simulink model "filters"  (R2025b)
settings: Solver=FixedStepDiscrete  StartTime=0.0  StopTime=inf  RelTol=1e-3
undefined symbols (not defined in the file or in its folder): Gain_rt
settings Model: Creator=linogarciamorales  LastModifiedBy=linogarciamorales
settings OptimizationCC: EnhancedBackFolding=on  PassReuseOutputArgsAs=Individual arguments  ZeroExternalMemoryAtStartup=off  ZeroInternalMemoryAtStartup=off  OptimizeBlockOrder=speed  DifferentSizesBufferReuse=on  OptimizationCustomize=off  EfficientTunableParamExpr=on
settings DebuggingCC: ParameterTunabilityLossMsg=error
settings HardwareCC: ProdBitPerPointer=32.0  ProdBitPerSizeT=32.0  ProdBitPerPtrDiffT=32.0  ProdLargestAtomicFloat=None  ProdIntDivRoundTo=Undefined  ProdEndianess=Unspecified  ProdWordSize=32.0  ProdHWDeviceType=Generic->32-bit Embedded Processor
settings SFSimCC: MATLABDynamicMemAlloc=off
settings RTWCC: SystemTargetFile=ert.tlc  GenCodeOnly=on  TemplateMakefile=ert_default_tmf  Description=Embedded Coder
settings CodeAppCC: ForceParamTrailComments=on  IgnoreCustomStorageClasses=off  OperatorAnnotations=on  SimulinkDataObjDesc=on  SFDataObjDesc=on  InsertBlockDesc=on
settings ERTTargetCC: InlinedParameterPlacement=Hierarchical  ERTCustomFileTemplate=example_file_process.tlc  TargetLangStandard=C99 (ISO)  SupportNonInlinedSFcns=on

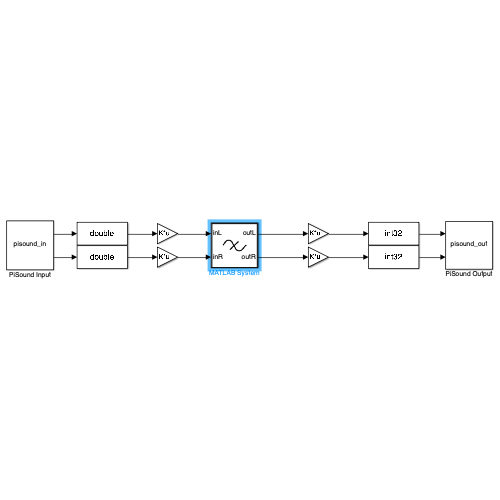
[thumbnail: Simulink's stored preview of the top-level diagram]
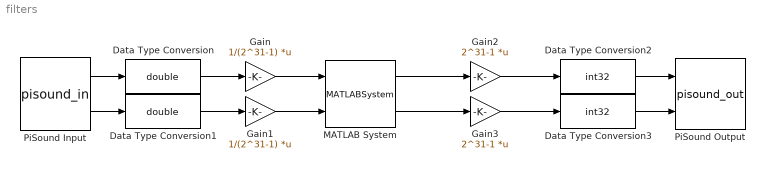
== system filters ==
  Data Type Conversion : DataTypeConversion  OutDataTypeStr=double  SaturateOnIntegerOverflow=off  RndMeth=Floor
  Data Type Conversion1 : DataTypeConversion  OutDataTypeStr=double  SaturateOnIntegerOverflow=off  RndMeth=Floor
  Data Type Conversion2 : DataTypeConversion  OutDataTypeStr=int32  SaturateOnIntegerOverflow=off  RndMeth=Floor
  Data Type Conversion3 : DataTypeConversion  OutDataTypeStr=int32  SaturateOnIntegerOverflow=off  RndMeth=Floor
  Gain : Gain  Gain=1/(2^31-1)  Multiplication=Matrix(K*u)
  Gain1 : Gain  Gain=1/(2^31-1)  Multiplication=Matrix(K*u)
  Gain2 : Gain  Gain=2^31-1  Multiplication=Matrix(K*u)
  Gain3 : Gain  Gain=2^31-1  Multiplication=Matrix(K*u)
  MATLAB System : MATLABSystem  InitFcn=|  System=filters_sys  N=128  Fs=48000  FilterType=FilterType_rt  Freq=Freq_rt  Q=Q_rt  Gain=Gain_rt  SimulateUsing=Code generation
      | Type_rt = uint8(1);   % 1..7
      | Freq_rt = 1000;       % Hz
      | Q_rt    = 0.707;
      | Gain_rt = 0;          % dB
      mask Type: filters_sys
  PiSound Input : S-Function  FunctionName=pisound_in  Parameters=48000, 128, 0  SFunctionDeploymentMode=off  EnableBusSupport=off
  PiSound Output : S-Function  FunctionName=pisound_out  Parameters=48000, 128, 0  SFunctionDeploymentMode=off  EnableBusSupport=off
  wires:
  PiSound Input/1 -> Data Type Conversion/1
  PiSound Input/2 -> Data Type Conversion1/1
  Data Type Conversion/1 -> Gain/1
  Data Type Conversion1/1 -> Gain1/1
  Gain2/1 -> Data Type Conversion2/1
  Gain3/1 -> Data Type Conversion3/1
  Gain/1 -> MATLAB System/1
  MATLAB System/1 -> Gain2/1
  Gain1/1 -> MATLAB System/2
  MATLAB System/2 -> Gain3/1
  Data Type Conversion2/1 -> PiSound Output/1
  Data Type Conversion3/1 -> PiSound Output/2
